simulink model "ponto3"  (R2018a)
settings: Solver=VariableStepAuto  StartTime=0.0  StopTime=100  RelTol=1e-3
values from neighbouring files (symbols this model uses):
  A_lqr = [A zeros(4, 1) ... (first row only)    [Model.m]
  B_lqr = [B ... (first row only)    [Model.m]
  C_lqr = eye(5)    [Model.m]
  D_lqr = zeros(5,2)    [Model.m]
  G0_inv = -([C_lqr(1,:);C_lqr(5,:)]*((A_lqr-B_lqr*Klqr)^(-1))*B_lqr*kuh)^(-1)    [Model.m]
  Klqr = lqr(A_lqr, B_lqr, Q, R)    [Model.m]
  kuh = [Klqr(:,1),Klqr(:,5)]    [Model.m]
settings Model: Creator=beapedroso  LastModifiedBy=tfesc

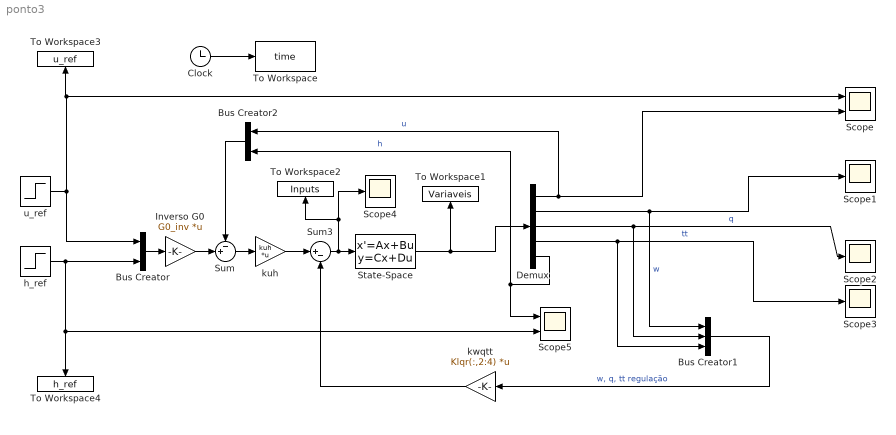
== system ponto3 ==
  Bus Creator : BusCreator  Inputs=2
  Bus Creator1 : BusCreator  Inputs=3
  Bus Creator2 : BusCreator  Inputs=2
  Clock : Clock
  Demux : Demux  Outputs=5
  Inverso G0 : Gain  Gain=G0_inv  Multiplication=Matrix(K*u)
  Scope : Scope  NumInputPorts=2
  Scope{1..4} (4 alike) : Scope
  Scope5 : Scope  NumInputPorts=2
  State-Space : StateSpace  A=A_lqr  B=B_lqr  C=C_lqr  D=D_lqr  InitialCondition=0
  Sum : Sum  Inputs=-+|
  Sum3 : Sum  Inputs=|+-
  To Workspace : ToWorkspace  VariableName=time  SampleTime=-1
  To Workspace1 : ToWorkspace  VariableName=Variaveis  SaveFormat=Structure With Time  SampleTime=0.1
  To Workspace2 : ToWorkspace  VariableName=Inputs  SaveFormat=Structure With Time  SampleTime=0.1
  To Workspace3 : ToWorkspace  VariableName=u_ref  SaveFormat=Structure With Time  SampleTime=0.1
  To Workspace4 : ToWorkspace  VariableName=h_ref  SaveFormat=Structure With Time  SampleTime=0.1
  "h_ref " : Step  After=10  SampleTime=50
  kuh : Gain  Gain=kuh  Multiplication=Matrix(K*u)
  kwqtt : Gain  Gain=Klqr(:,2:4)  Multiplication=Matrix(K*u)
  u_ref : Step  After=3  SampleTime=0
  wires:
  State-Space/1 -> Demux/1, To Workspace1/1
  Demux/2 -> Scope1/1, Bus Creator1/1  "w"
  Demux/3 -> Scope2/1, Bus Creator1/2  "q"
  Bus Creator1/1 -> kwqtt/1  "w, q, tt regulação"
  u_ref/1 -> Bus Creator/1, To Workspace3/1, Scope/1
  Clock/1 -> To Workspace/1
  Demux/5 -> Bus Creator2/2, Scope5/1  "h"
  Demux/4 -> Scope3/1, Bus Creator1/3  "tt"
  kwqtt/1 -> Sum3/2
  "h_ref "/1 -> Bus Creator/2, Scope5/2, To Workspace4/1
  Bus Creator/1 -> Inverso G0/1
  Inverso G0/1 -> Sum/2
  Demux/1 -> Bus Creator2/1, Scope/2  "u"
  Sum3/1 -> Scope4/1, To Workspace2/1, State-Space/1
  kuh/1 -> Sum3/1
  Bus Creator2/1 -> Sum/1
  Sum/1 -> kuh/1
